simulink model "progetto_ese3_sim"  (R2024a)
settings: Solver=VariableStepAuto  StartTime=0.0  StopTime=4  RelTol=1e-3
values from neighbouring files (symbols this model uses):
  Alin = J1    [progetto_ese3.m]
  Blin = double(subs(jacobian(f,u),[x1,x2,u],[xeq1,ueq]))    [progetto_ese3.m]
  Clin1 = double(subs(jacobian(g1,[x1,x2]),[x1,x2,u],[xeq1,ueq]))    [progetto_ese3.m]
  Clin2 = double(subs(jacobian(g2,[x1,x2]),[x1,x2,u],[xeq1,ueq]))    [progetto_ese3.m]
  ueq = 0    [progetto_ese3.m]
settings Model: Creator=USER  LastModifiedBy=USER
settings RTWCC: GPUComputeCapability=3.5

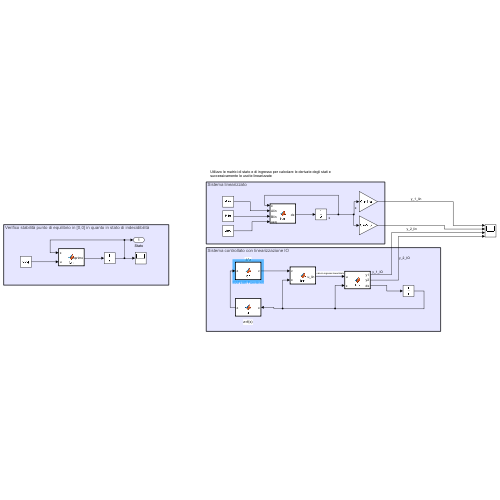
[thumbnail: Simulink's stored preview of the top-level diagram]
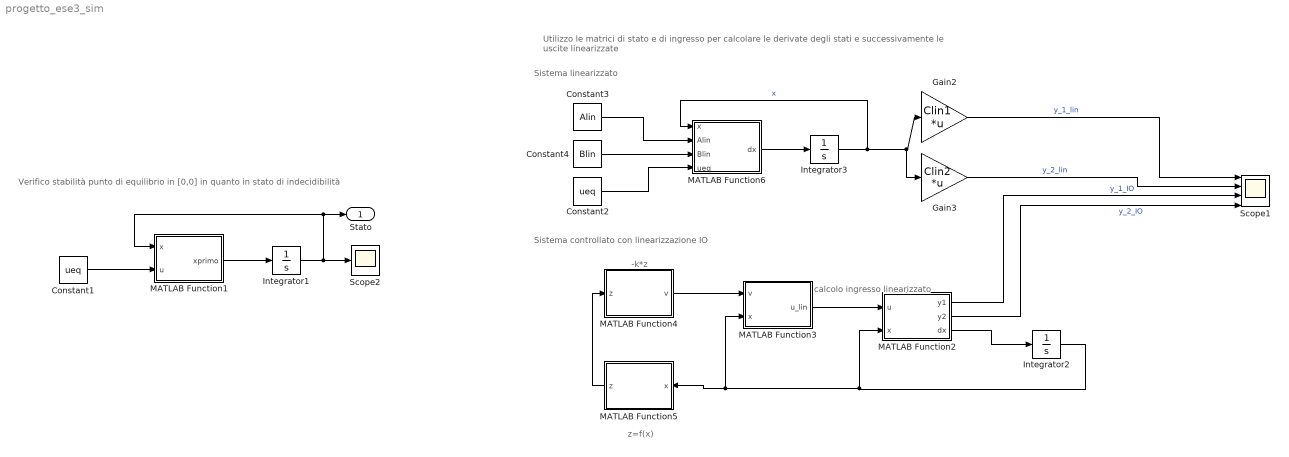
== system progetto_ese3_sim ==
  note: -k*z
  note: z=f(x)
  note: calcolo ingresso linearizzato
  note: Utilizzo le matrici di stato e di ingresso per calcolare le derivate degli stati e successivamente le uscite linearizzate
  note: Sistema controllato con linearizzazione IO
  note: Sistema linearizzato
  note: Verifico stabilità punto di equilibrio in [0,0] in quanto in stato di indecidibilità
  Constant1 : Constant  Value=ueq
  Constant2 : Constant  Value=ueq
  Constant3 : Constant  Value=Alin
  Constant4 : Constant  Value=Blin
  Gain2 : Gain  Gain=Clin1  Multiplication=Matrix(K*u)
  Gain3 : Gain  Gain=Clin2  Multiplication=Matrix(K*u)
  Integrator1 : Integrator  InitialCondition=[-0.1;0.1]
  Integrator2 : Integrator  InitialCondition=[3;5]
  Integrator3 : Integrator  InitialCondition=[3;5]
  MATLAB Function1 : MATLAB Function  TreatAsAtomicUnit=on
  MATLAB Function2 : MATLAB Function  TreatAsAtomicUnit=on
  MATLAB Function3 : MATLAB Function  TreatAsAtomicUnit=on
  MATLAB Function4 : MATLAB Function  TreatAsAtomicUnit=on
  MATLAB Function5 : MATLAB Function  TreatAsAtomicUnit=on
  MATLAB Function6 : MATLAB Function  TreatAsAtomicUnit=on
  Scope1 : Scope  NumInputPorts=4
  Scope2 : Scope
  Stato : Outport
  wires:
  Constant1/1 -> MATLAB Function1/2(u)
  MATLAB Function1/1(xprimo) -> Integrator1/1
  Integrator1/1 -> Scope2/1, MATLAB Function1/1(x), Stato/1
  MATLAB Function2/2(y2) -> Scope1/4  "y_2_IO"
  MATLAB Function4/1(v) -> MATLAB Function3/1(v)
  MATLAB Function3/1(u_lin) -> MATLAB Function2/1(u)
  Integrator2/1 -> MATLAB Function2/2(x), MATLAB Function3/2(x), MATLAB Function5/1(x)
  MATLAB Function5/1(z) -> MATLAB Function4/1(z)
  MATLAB Function2/3(dx) -> Integrator2/1
  MATLAB Function2/1(y1) -> Scope1/3  "y_1_IO"
  Integrator3/1 -> Gain3/1, Gain2/1, MATLAB Function6/1(x)  "x"
  Gain3/1 -> Scope1/2  "y_2_lin"
  Constant2/1 -> MATLAB Function6/4(ueq)
  Constant4/1 -> MATLAB Function6/3(Blin)
  Constant3/1 -> MATLAB Function6/2(Alin)
  MATLAB Function6/1(dx) -> Integrator3/1
  Gain2/1 -> Scope1/1  "y_1_lin"

== matlab function progetto_ese3_sim/MATLAB Function1 ==
  data: x input; u input; xprimo output
function xprimo = fcn(x,u)
x1=x(1);
x2=x(2);
u=0;
xprimo = [ 3*(x1.^2+x1).*x2;
          -4.*x2+x1-x2.*u+3.*u];

== matlab function progetto_ese3_sim/MATLAB Function2 ==
  data: y1 output; y2 output; u input; dx output; x input
function [y1,y2,dx] = fcn(u,x)

x1 = x(1);
x2 = x(2);
dx = [3*(x1^2+x1)*x2; -4*x2+x1-x2*u+3*u];
y1 = 5*x2;
y2 = 2*x1;

== matlab function progetto_ese3_sim/MATLAB Function3 ==
  data: u_lin output; v input; x input
function u_lin  = fcn(v,x)

x1 = x(1);
x2 = x(2);
u_lin =  ((6*x1^2 + 6*x1)*(x1 - 4*x2)- v + 2*x2^2*(6*x1 + 3)*(3*x1^2 + 3*x1))/((6*x1^2 + 6*x1)*(x2 - 3));

== matlab function progetto_ese3_sim/MATLAB Function4 ==
  data: v output; z input
function v  = fcn(z)

z1 = z(1);
z2 = z(2);
K = [12.5,7.5];
v = -K(1)*z1-K(2)*z2; % -K*z

== matlab function progetto_ese3_sim/MATLAB Function5 ==
  data: z output; x input
function z  = fcn(x)

x1 = x(1);
x2 = x(2);
z = [2*x1; 2*x2*(3*x1^2 + 3*x1)];

== matlab function progetto_ese3_sim/MATLAB Function6 ==
  data: x input; Alin input; Blin input; ueq input; dx output
function dx = fcn(x, Alin, Blin, ueq)


dx = Alin*x +Blin*ueq;
